simulink model "quad_simtest"  (R2023b)
settings: Solver=ode1  StartTime=0.0  StopTime=100  FixedStep=0.0001  RelTol=1e-3
libraries: uavutilslib x1
settings Model: Creator=soemt  LastModifiedBy=soemt

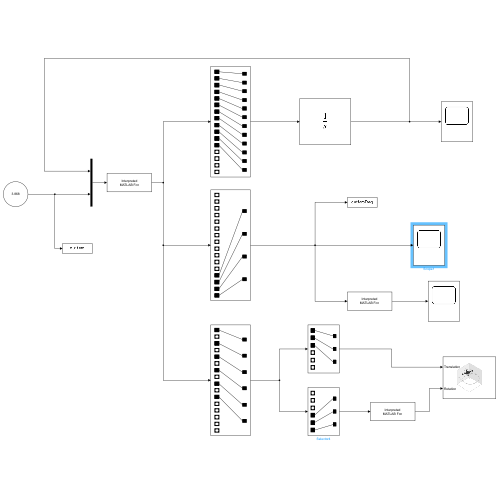
[thumbnail: Simulink's stored preview of the top-level diagram]
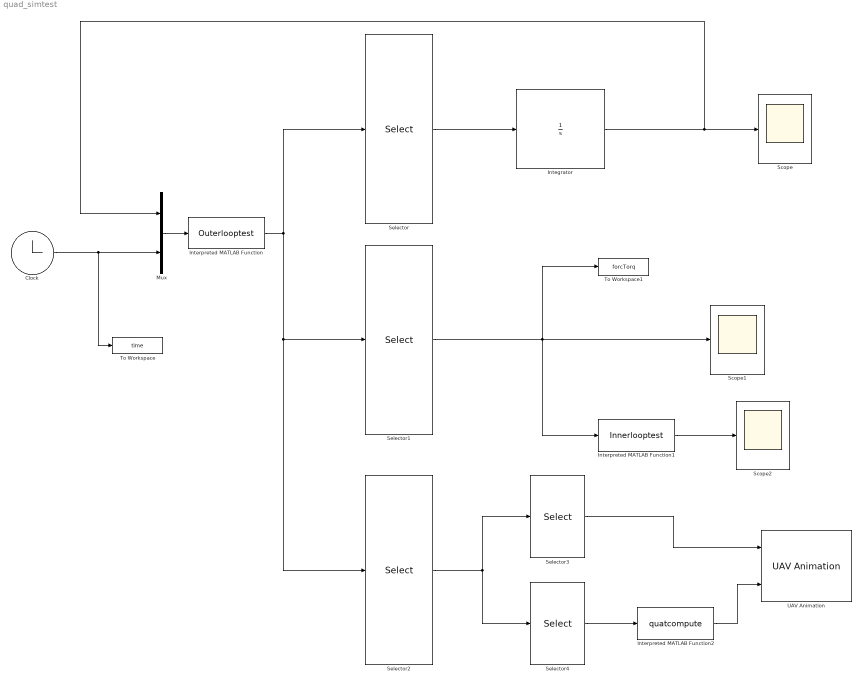
== system quad_simtest ==
  Clock : Clock
  Integrator : Integrator  InitialCondition=[1 0 -1 0 0 0 0.1 0 -0.2 0 0.2 0]
  Interpreted MATLAB Function : MATLABFcn  MATLABFcn=Outerlooptest  OutputDimensions=16
  Interpreted MATLAB Function1 : MATLABFcn  MATLABFcn=Innerlooptest  OutputDimensions=4
  Interpreted MATLAB Function2 : MATLABFcn  MATLABFcn=quatcompute  OutputDimensions=4
  Mux : Mux  Inputs=2
  Scope : Scope
  Scope1 : Scope
  Scope2 : Scope
  Selector : Selector  InputPortWidth=16  IndexOptions=Index vector (dialog)  Indices=[1 2 3 4 5 6 7 8 9 10 11 12]  OutputSizes=1
  Selector1 : Selector  InputPortWidth=16  IndexOptions=Index vector (dialog)  Indices=[13 14 15 16]  OutputSizes=1
  Selector2 : Selector  InputPortWidth=16  IndexOptions=Index vector (dialog)  Indices=[1 3 5 7 9 11]  OutputSizes=1
  Selector3 : Selector  InputPortWidth=6  IndexOptions=Index vector (dialog)  Indices=[1 2 3]  OutputSizes=1
  Selector4 : Selector  InputPortWidth=6  IndexOptions=Index vector (dialog)  Indices=[4 5 6]  OutputSizes=1
  To Workspace : ToWorkspace  VariableName=time  SampleTime=-1
  To Workspace1 : ToWorkspace  VariableName=forcTorq  SampleTime=-1
  UAV Animation : uavutilslib/UAV Animation  UAVType=Multirotor  UAVSize=1  InertialZDirection=Up  SampleTime=-1
  wires:
  Clock/1 -> Mux/2, To Workspace/1
  Mux/1 -> Interpreted MATLAB Function/1
  Interpreted MATLAB Function/1 -> Selector/1, Selector2/1, Selector1/1
  Selector/1 -> Integrator/1
  Integrator/1 -> Mux/1, Scope/1
  Selector1/1 -> Interpreted MATLAB Function1/1, To Workspace1/1, Scope1/1
  Interpreted MATLAB Function1/1 -> Scope2/1
  Selector2/1 -> Selector3/1, Selector4/1
  Selector4/1 -> Interpreted MATLAB Function2/1
  Interpreted MATLAB Function2/1 -> UAV Animation/2
  Selector3/1 -> UAV Animation/1
